simulink model "eovsa_corr_300mhz"  (R2012b)
settings: Solver=VariableStepDiscrete  SolverMode=SingleTasking  StartTime=0.0  StopTime=5000  RelTol=1e-3
undefined symbols (not defined in the file or in its folder): A, B, gcbh, PCIN, sfp, xlBlockLoadCallback, xlipgetpartsetting
libraries: xbsIndex_r4 x5996, casper_library_misc x52, simulink x33, dspsigops x24, xps_library x15, casper_library_delays x2
(part 6 of 65)

== system eovsa_corr_300mhz/packet_buffer0 ==
  note: TODO: Clean up some no longer used logic.
  din : Inport
  dvalid : Inport  Port=2
  eof : Inport  Port=3
  hdr : Inport  Port=4
  hdr_valid : Inport  Port=5
  rd_addr_in : Inport  Port=6
  rd_valid_in : Inport  Port=7
  Convert3 : xbsIndex_r4/Convert  gui_display_data_type=Fixed-point  arith_type=Unsigned  n_bits=n_boards  bin_pt=0  float_type=Single  exp_bits=8  fraction_bits=24  quantization=Truncate  overflow=Wrap  en=off  latency=0  dbl_ovrd=off  pipeline=off  block_type=convert
      settings: block_version=11.4
  Delay{1,3,5,7..10,15..17,19..20,22..25} (16 alike) : xbsIndex_r4/Delay  rst=off  infoeditControl=Selection of Reset will increase slice count due to use of real FFs and instead of SRLs  en=off  latency=1  dbl_ovrd=off  reg_retiming=on  block_type=delay
      settings: block_version=11.4
  Delay4 : xbsIndex_r4/Delay  rst=off  infoeditControl=Selection of Reset will increase slice count due to use of real FFs and instead of SRLs  en=on  latency=1  dbl_ovrd=off  reg_retiming=on  block_type=delay
      settings: block_version=11.4
  Logical : xbsIndex_r4/Logical  logical_function=AND  inputs=2  en=off  latency=0  precision=Full  arith_type=Unsigned  n_bits=16  bin_pt=0  align_bp=on  dbl_ovrd=off  block_type=logical
  Slice1 : xbsIndex_r4/Slice  nbits=16  boolean_output=off  mode=Lower Bit Location + Width  bit1=0  base1=MSB of Input  bit0=0  base0=LSB of Input  dbl_ovrd=off  block_type=slice
  Slice3 : xbsIndex_r4/Slice  nbits=48  boolean_output=off  mode=Upper Bit Location + Width  bit1=0  base1=MSB of Input  bit0=0  base0=LSB of Input  dbl_ovrd=off  block_type=slice
  Slice5 : xbsIndex_r4/Slice  nbits=freq_chan - (n_boards + n_x)  boolean_output=off  mode=Lower Bit Location + Width  bit1=0  base1=MSB of Input  bit0=16  base0=LSB of Input  dbl_ovrd=off  block_type=slice
  buffer0 : Subsystem
  word_counter : xbsIndex_r4/Counter  cnt_type=Free Running  cnt_to=Inf  operation=Up  start_count=0  cnt_by_val=1  arith_type=Unsigned  n_bits=pkt_len  bin_pt=0  load_pin=off  rst=on  en=on  explicit_period=off  period=1  dbl_ovrd=off  use_behavioral_HDL=off  implementation=Fabric  block_type=counter
      settings: block_version=11.4
  sync : Outport
  d0 : Outport  Port=2
  dv0 : Outport  Port=3
  mcnt_out0 : Outport  Port=4
  rd_addr_out : Outport  Port=5
  rd_valid_out0 : Outport  Port=6
  rd_valid_out1 : Outport  Port=7
  wires:
  Delay15/1 -> [din]
  Delay9/1 -> [word]
  Delay8/1 -> [ant]
  Delay5/1 -> [freq]
  Delay3/1 -> [we]
  Delay1/1 -> [mcnt]
  Convert3/1 -> Delay22/1
  Delay23/1 -> Delay1/1
  Slice5/1 -> Delay16/1
  Delay22/1 -> Delay8/1
  Delay17/1 -> Delay9/1
  Delay16/1 -> Delay5/1
  Delay10/1 -> Delay15/1
  din/1 -> Delay10/1
  Delay7/1 -> Delay3/1
  hdr_valid/1 -> Delay4/2
  Delay4/1 -> Slice5/1, Slice3/1, Slice1/1
  hdr/1 -> Delay4/1
  dvalid/1 -> Logical/1, word_counter/2, Delay7/1
  buffer0/4(mcnt) -> mcnt_out0/1
  buffer0/3(dout_valid) -> dv0/1
  buffer0/2(dout) -> d0/1
  buffer0/1(sync) -> sync/1
  word_counter/1 -> Delay17/1
  Slice3/1 -> Delay23/1
  Slice1/1 -> Convert3/1
  [din] -> buffer0/1(data)
  [freq] -> buffer0/2(freq)
  [we] -> buffer0/3(dvalid)
  [ant] -> buffer0/4(ant)
  [word] -> buffer0/5(word)
  [mcnt] -> buffer0/6(mcnt_in)
  buffer0/6(rd_valid_out0) -> rd_valid_out0/1
  buffer0/5(rd_addr_out) -> rd_addr_out/1
  Delay20/1 -> [rd_addr_in]
  Delay19/1 -> Delay20/1
  Delay25/1 -> [rd_valid_in]
  Delay24/1 -> Delay25/1
  rd_addr_in/1 -> Delay19/1
  rd_valid_in/1 -> Delay24/1
  [rd_addr_in] -> buffer0/7(rd_addr_in)
  [rd_valid_in] -> buffer0/8(rd_valid_in)
  Logical/1 -> word_counter/1
  eof/1 -> Logical/2
  buffer0/7(rd_valid_out1) -> rd_valid_out1/1

== system eovsa_corr_300mhz/packet_buffer1 ==
  note: TODO: Clean up some no longer used logic.
  din : Inport
  dvalid : Inport  Port=2
  eof : Inport  Port=3
  hdr : Inport  Port=4
  hdr_valid : Inport  Port=5
  rd_addr_in : Inport  Port=6
  rd_valid_in : Inport  Port=7
  Convert3 : xbsIndex_r4/Convert  gui_display_data_type=Fixed-point  arith_type=Unsigned  n_bits=n_boards  bin_pt=0  float_type=Single  exp_bits=8  fraction_bits=24  quantization=Truncate  overflow=Wrap  en=off  latency=0  dbl_ovrd=off  pipeline=off  block_type=convert
      settings: block_version=11.4
  Delay{1,3,5,7..10,15..17,19..20,22..25} (16 alike) : xbsIndex_r4/Delay  rst=off  infoeditControl=Selection of Reset will increase slice count due to use of real FFs and instead of SRLs  en=off  latency=1  dbl_ovrd=off  reg_retiming=on  block_type=delay
      settings: block_version=11.4
  Delay4 : xbsIndex_r4/Delay  rst=off  infoeditControl=Selection of Reset will increase slice count due to use of real FFs and instead of SRLs  en=on  latency=1  dbl_ovrd=off  reg_retiming=on  block_type=delay
      settings: block_version=11.4
  Logical : xbsIndex_r4/Logical  logical_function=AND  inputs=2  en=off  latency=0  precision=Full  arith_type=Unsigned  n_bits=16  bin_pt=0  align_bp=on  dbl_ovrd=off  block_type=logical
  Slice1 : xbsIndex_r4/Slice  nbits=16  boolean_output=off  mode=Lower Bit Location + Width  bit1=0  base1=MSB of Input  bit0=0  base0=LSB of Input  dbl_ovrd=off  block_type=slice
  Slice3 : xbsIndex_r4/Slice  nbits=48  boolean_output=off  mode=Upper Bit Location + Width  bit1=0  base1=MSB of Input  bit0=0  base0=LSB of Input  dbl_ovrd=off  block_type=slice
  Slice5 : xbsIndex_r4/Slice  nbits=freq_chan - (n_boards + n_x)  boolean_output=off  mode=Lower Bit Location + Width  bit1=0  base1=MSB of Input  bit0=16  base0=LSB of Input  dbl_ovrd=off  block_type=slice
  buffer0 : Subsystem
  word_counter : xbsIndex_r4/Counter  cnt_type=Free Running  cnt_to=Inf  operation=Up  start_count=0  cnt_by_val=1  arith_type=Unsigned  n_bits=pkt_len  bin_pt=0  load_pin=off  rst=on  en=on  explicit_period=off  period=1  dbl_ovrd=off  use_behavioral_HDL=off  implementation=Fabric  block_type=counter
      settings: block_version=11.4
  sync : Outport
  d0 : Outport  Port=2
  dv0 : Outport  Port=3
  mcnt_out0 : Outport  Port=4
  rd_addr_out : Outport  Port=5
  rd_valid_out0 : Outport  Port=6
  rd_valid_out1 : Outport  Port=7
  wires:
  buffer0/7(rd_valid_out1) -> rd_valid_out1/1
  eof/1 -> Logical/2
  Logical/1 -> word_counter/1
  [rd_valid_in] -> buffer0/8(rd_valid_in)
  [rd_addr_in] -> buffer0/7(rd_addr_in)
  rd_valid_in/1 -> Delay24/1
  rd_addr_in/1 -> Delay19/1
  Delay24/1 -> Delay25/1
  Delay25/1 -> [rd_valid_in]
  Delay19/1 -> Delay20/1
  Delay20/1 -> [rd_addr_in]
  buffer0/5(rd_addr_out) -> rd_addr_out/1
  buffer0/6(rd_valid_out0) -> rd_valid_out0/1
  [mcnt] -> buffer0/6(mcnt_in)
  [word] -> buffer0/5(word)
  [ant] -> buffer0/4(ant)
  [we] -> buffer0/3(dvalid)
  [freq] -> buffer0/2(freq)
  [din] -> buffer0/1(data)
  Slice1/1 -> Convert3/1
  Slice3/1 -> Delay23/1
  word_counter/1 -> Delay17/1
  buffer0/1(sync) -> sync/1
  buffer0/2(dout) -> d0/1
  buffer0/3(dout_valid) -> dv0/1
  buffer0/4(mcnt) -> mcnt_out0/1
  dvalid/1 -> Delay7/1, word_counter/2, Logical/1
  hdr/1 -> Delay4/1
  Delay4/1 -> Slice1/1, Slice3/1, Slice5/1
  hdr_valid/1 -> Delay4/2
  Delay7/1 -> Delay3/1
  din/1 -> Delay10/1
  Delay10/1 -> Delay15/1
  Delay16/1 -> Delay5/1
  Delay17/1 -> Delay9/1
  Delay22/1 -> Delay8/1
  Slice5/1 -> Delay16/1
  Delay23/1 -> Delay1/1
  Convert3/1 -> Delay22/1
  Delay1/1 -> [mcnt]
  Delay3/1 -> [we]
  Delay5/1 -> [freq]
  Delay8/1 -> [ant]
  Delay9/1 -> [word]
  Delay15/1 -> [din]

== system eovsa_corr_300mhz/packet_count_p ==
  out_reg : Inport
  assert_reg : xbsIndex_r4/Assert  assert_type=on  type_source=Explicitly  gui_display_data_type=Fixed-point  arith_type=Unsigned  n_bits=32  bin_pt=0  preci_type=Single  exp_width=8  frac_width=24  assert_rate=off  rate_source=Explicitly  period=1  output_port=on  block_type=assert
  cast_gw : xbsIndex_r4/Convert  gui_display_data_type=Fixed-point  arith_type=Unsigned  n_bits=32  bin_pt=0  float_type=Single  exp_bits=8  fraction_bits=24  quantization=Truncate  overflow=Wrap  en=off  latency=0  dbl_ovrd=off  pipeline=off  block_type=convert
  eovsa_corr_300mhz_packet_count_p_user_data_in : xbsIndex_r4/Gateway Out  inherit_from_input=off  hdl_port=on  timing_constraint=None  locs_specified=off  LOCs={}  UseAsDAC=off  DACChannel='1'  block_type=gatewayout
  io_delay : xbsIndex_r4/Delay  rst=off  infoeditControl=Selection of Reset will increase slice count due to use of real FFs and instead of SRLs  en=off  latency=0  dbl_ovrd=off  reg_retiming=on  block_type=delay
  reint1 : xbsIndex_r4/Reinterpret  force_arith_type=on  arith_type=Unsigned  force_bin_pt=on  bin_pt=0  block_type=reinterpret
  sim_out : Outport
  wires:
  io_delay/1 -> cast_gw/1
  cast_gw/1 -> eovsa_corr_300mhz_packet_count_p_user_data_in/1
  eovsa_corr_300mhz_packet_count_p_user_data_in/1 -> sim_out/1
  out_reg/1 -> assert_reg/1
  assert_reg/1 -> reint1/1
  reint1/1 -> io_delay/1

== system eovsa_corr_300mhz/packet_count_x ==
  out_reg : Inport
  assert_reg : xbsIndex_r4/Assert  assert_type=on  type_source=Explicitly  gui_display_data_type=Fixed-point  arith_type=Unsigned  n_bits=32  bin_pt=0  preci_type=Single  exp_width=8  frac_width=24  assert_rate=off  rate_source=Explicitly  period=1  output_port=on  block_type=assert
  cast_gw : xbsIndex_r4/Convert  gui_display_data_type=Fixed-point  arith_type=Unsigned  n_bits=32  bin_pt=0  float_type=Single  exp_bits=8  fraction_bits=24  quantization=Truncate  overflow=Wrap  en=off  latency=0  dbl_ovrd=off  pipeline=off  block_type=convert
  eovsa_corr_300mhz_packet_count_x_user_data_in : xbsIndex_r4/Gateway Out  inherit_from_input=off  hdl_port=on  timing_constraint=None  locs_specified=off  LOCs={}  UseAsDAC=off  DACChannel='1'  block_type=gatewayout
  io_delay : xbsIndex_r4/Delay  rst=off  infoeditControl=Selection of Reset will increase slice count due to use of real FFs and instead of SRLs  en=off  latency=0  dbl_ovrd=off  reg_retiming=on  block_type=delay
  reint1 : xbsIndex_r4/Reinterpret  force_arith_type=on  arith_type=Unsigned  force_bin_pt=on  bin_pt=0  block_type=reinterpret
  sim_out : Outport
  wires:
  io_delay/1 -> cast_gw/1
  cast_gw/1 -> eovsa_corr_300mhz_packet_count_x_user_data_in/1
  eovsa_corr_300mhz_packet_count_x_user_data_in/1 -> sim_out/1
  out_reg/1 -> assert_reg/1
  assert_reg/1 -> reint1/1
  reint1/1 -> io_delay/1

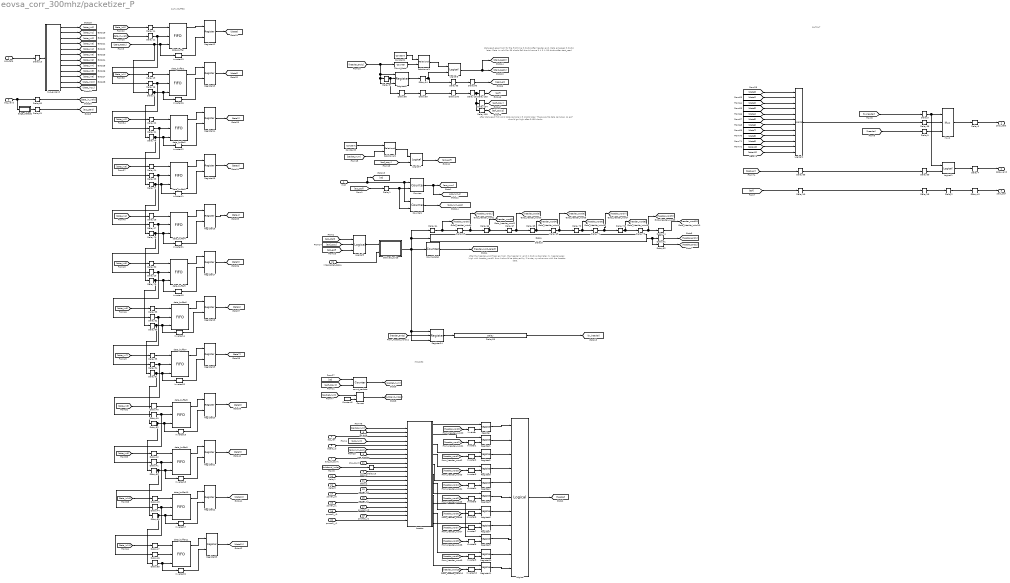
== system eovsa_corr_300mhz/packetizer_P ==
  note: After the header_word flags go high, the header is valid 2 clock cycles later.
      | tx_header goes high with header_word0, thus it should be delayed by 2 to stay synchronous with the header data.
  note: after start_read first valid data sample is 3 clocks later.
      | There are 96 data samples, so eof should go high after 3+95 clocks
  note: start_read goes high for the first time 3 clocks after header_end.
      | Data emerges 3 clocks later.
      | Data is valid for 96 clocks
      | Eof should come 3 + 3 + 95 clocks after start_read
  note: OUTPUT
  note: HEADER
  note: DATA BUFFER
  mrst : Inport
  acc_data : Inport  Port=2
  acc_valid : Inport  Port=3
  acc_len : Inport  Port=4
  use_circular : Inport  Port=5
  board_id : Inport  Port=6
  adc_of_count : Inport  Port=7
  fft_shift : Inport  Port=8
  delay0 : Inport  Port=9
  delay1 : Inport  Port=10
  delay2 : Inport  Port=11
  delay3 : Inport  Port=12
  power_x0 : Inport  Port=13
  power_y0 : Inport  Port=14
  power_x1 : Inport  Port=15
  power_y1 : Inport  Port=16
  power2_x0 : Inport  Port=17
  power2_y0 : Inport  Port=18
  power2_x1 : Inport  Port=19
  power2_y1 : Inport  Port=20
  clip_count : Inport  Port=21
  interpacket_delay : Inport  Port=22
  Concat : xbsIndex_r4/Concat  num_inputs=2  dbl_ovrd=off  block_type=concat
  Constant1 : xbsIndex_r4/Constant  const=0  gui_display_data_type=Fixed-point  arith_type=Unsigned  n_bits=4  bin_pt=0  preci_type=Single  exp_width=8  frac_width=24  explicit_period=on  period=1  equ=P=C  opselect=C  inp2=PCIN>>17  opr=+  inp1=P  carry=CIN  dbl_ovrd=off  block_type=constant
      settings: block_version=11.4
  Constant2 : xbsIndex_r4/Constant  const=0  gui_display_data_type=Fixed-point  arith_type=Unsigned  n_bits=log2( (2 ^ freq_chan) / n_packets )  bin_pt=0  preci_type=Single  exp_width=8  frac_width=24  explicit_period=on  period=1  equ=P=C  opselect=C  inp2=PCIN>>17  opr=+  inp1=P  carry=CIN  dbl_ovrd=off  block_type=constant
      settings: block_version=11.4
  Constant3 : xbsIndex_r4/Constant  const=n_packets - 1  gui_display_data_type=Fixed-point  arith_type=Unsigned  n_bits=ceil( log2( n_packets - 1 ) )  bin_pt=0  preci_type=Single  exp_width=8  frac_width=24  explicit_period=on  period=1  equ=P=C  opselect=C  inp2=PCIN>>17  opr=+  inp1=P  carry=CIN  dbl_ovrd=off  block_type=constant
      settings: block_version=11.4
  Count_data1 : xbsIndex_r4/Counter  cnt_type=Count Limited  cnt_to=header_len / 8 - 1  operation=Up  start_count=0  cnt_by_val=1  arith_type=Unsigned  n_bits=ceil( log2( header_len / 8 - 1 ) )  bin_pt=0  load_pin=off  rst=on  en=off  explicit_period=on  period=1  dbl_ovrd=off  use_behavioral_HDL=on  implementation=Fabric  use_rpm=off  block_type=counter
  Count_data7 : xbsIndex_r4/Counter  cnt_type=Count Limited  cnt_to=11  operation=Up  start_count=0  cnt_by_val=1  arith_type=Unsigned  n_bits=4  bin_pt=0  load_pin=off  rst=on  en=off  explicit_period=on  period=1  dbl_ovrd=off  use_behavioral_HDL=on  implementation=Fabric  use_rpm=off  block_type=counter
  Counter : xbsIndex_r4/Counter  cnt_type=Free Running  cnt_to=Inf  operation=Up  start_count=0  cnt_by_val=1  arith_type=Unsigned  n_bits=32  bin_pt=0  load_pin=off  rst=on  en=on  explicit_period=off  period=1  dbl_ovrd=off  use_behavioral_HDL=off  implementation=DSP48  block_type=counter
      settings: block_version=11.4
  Counter1 : xbsIndex_r4/Counter  cnt_type=Count Limited  cnt_to=49  operation=Up  start_count=0  cnt_by_val=1  arith_type=Unsigned  n_bits=8  bin_pt=0  load_pin=off  rst=on  en=on  explicit_period=off  period=1  dbl_ovrd=off  use_behavioral_HDL=off  implementation=Fabric  block_type=counter
      settings: block_version=11.4
  Delay{1..4,6,9,13..14,32,34,41,43..44,48..49,56,58..59,64..74,95,98..100} (33 alike) : xbsIndex_r4/Delay  rst=off  infoeditControl=Selection of Reset will increase slice count due to use of real FFs and instead of SRLs  en=off  latency=1  dbl_ovrd=off  reg_retiming=on  block_type=delay
      settings: block_version=11.4
  Delay{7,11,15..16,21,23,27,29,39,46,60..61,76..85,91..92,94,102..105} (29 alike) : xbsIndex_r4/Delay  rst=off  infoeditControl=Selection of Reset will increase slice count due to use of real FFs and instead of SRLs  en=off  latency=1  dbl_ovrd=off  reg_retiming=off  block_type=delay
      settings: block_version=11.4
  Delay19 : xbsIndex_r4/Delay  rst=off  infoeditControl=Selection of Reset will increase slice count due to use of real FFs and instead of SRLs  en=off  latency=2  dbl_ovrd=off  reg_retiming=on  block_type=delay
      settings: block_version=11.4
  Delay22 : xbsIndex_r4/Delay  rst=off  infoeditControl=Selection of Reset will increase slice count due to use of real FFs and instead of SRLs  en=off  latency=3  dbl_ovrd=off  reg_retiming=on  block_type=delay
      settings: block_version=11.4
  Delay24 : xbsIndex_r4/Delay  rst=off  infoeditControl=Selection of Reset will increase slice count due to use of real FFs and instead of SRLs  en=off  latency=4  dbl_ovrd=off  reg_retiming=on  block_type=delay
      settings: block_version=11.4
  Delay28 : xbsIndex_r4/Delay  rst=off  infoeditControl=Selection of Reset will increase slice count due to use of real FFs and instead of SRLs  en=off  latency=5  dbl_ovrd=off  reg_retiming=on  block_type=delay
      settings: block_version=11.4
  Delay30 : xbsIndex_r4/Delay  rst=off  infoeditControl=Selection of Reset will increase slice count due to use of real FFs and instead of SRLs  en=off  latency=6  dbl_ovrd=off  reg_retiming=on  block_type=delay
      settings: block_version=11.4
  Delay33 : xbsIndex_r4/Delay  rst=off  infoeditControl=Selection of Reset will increase slice count due to use of real FFs and instead of SRLs  en=off  latency=7  dbl_ovrd=off  reg_retiming=on  block_type=delay
      settings: block_version=11.4
  Delay35 : xbsIndex_r4/Delay  rst=off  infoeditControl=Selection of Reset will increase slice count due to use of real FFs and instead of SRLs  en=off  latency=8  dbl_ovrd=off  reg_retiming=on  block_type=delay
      settings: block_version=11.4
  Delay40 : xbsIndex_r4/Delay  rst=off  infoeditControl=Selection of Reset will increase slice count due to use of real FFs and instead of SRLs  en=off  latency=9  dbl_ovrd=off  reg_retiming=on  block_type=delay
      settings: block_version=11.4
  Delay42 : xbsIndex_r4/Delay  rst=off  infoeditControl=Selection of Reset will increase slice count due to use of real FFs and instead of SRLs  en=off  latency=10  dbl_ovrd=off  reg_retiming=on  block_type=delay
      settings: block_version=11.4
  Delay45 : xbsIndex_r4/Delay  rst=off  infoeditControl=Selection of Reset will increase slice count due to use of real FFs and instead of SRLs  en=off  latency=11  dbl_ovrd=off  reg_retiming=on  block_type=delay
      settings: block_version=11.4
  Delay47 : xbsIndex_r4/Delay  rst=off  infoeditControl=Selection of Reset will increase slice count due to use of real FFs and instead of SRLs  en=off  latency=12  dbl_ovrd=off  reg_retiming=on  block_type=delay
      settings: block_version=11.4
  Delay5 : xbsIndex_r4/Delay  rst=off  infoeditControl=Selection of Reset will increase slice count due to use of real FFs and instead of SRLs  en=off  latency=10  dbl_ovrd=off  reg_retiming=on  block_type=delay
      settings: block_version=11.4
  Delay53 : xbsIndex_r4/Delay  rst=off  infoeditControl=Selection of Reset will increase slice count due to use of real FFs and instead of SRLs  en=off  latency=2  dbl_ovrd=off  reg_retiming=on  block_type=delay
      settings: block_version=11.4
  Delay96 : xbsIndex_r4/Delay  rst=off  infoeditControl=Selection of Reset will increase slice count due to use of real FFs and instead of SRLs  en=off  latency=3  dbl_ovrd=off  reg_retiming=on  block_type=delay
      settings: block_version=11.4
  Delay97 : xbsIndex_r4/Delay  rst=off  infoeditControl=Selection of Reset will increase slice count due to use of real FFs and instead of SRLs  en=off  latency=data_len / 8  dbl_ovrd=off  reg_retiming=off  block_type=delay
      settings: block_version=11.4
  Inverter{,1..10} (11 alike) : xbsIndex_r4/Inverter  en=off  latency=0  dbl_ovrd=off  block_type=inv
  Inverter{11..22} (12 alike) : xbsIndex_r4/Inverter  en=off  latency=2  dbl_ovrd=off  block_type=inv
  Logical : xbsIndex_r4/Logical  logical_function=OR  inputs=11  en=off  latency=1  precision=Full  arith_type=Unsigned  n_bits=16  bin_pt=0  align_bp=on  dbl_ovrd=off  block_type=logical
  Logical1 : xbsIndex_r4/Logical  logical_function=OR  inputs=2  en=off  latency=1  precision=Full  arith_type=Unsigned  n_bits=16  bin_pt=0  align_bp=on  dbl_ovrd=off  block_type=logical
      settings: block_version=11.4
  Logical2 : xbsIndex_r4/Logical  logical_function=OR  inputs=12  en=off  latency=1  precision=Full  arith_type=Unsigned  n_bits=16  bin_pt=0  align_bp=on  dbl_ovrd=off  block_type=logical
  Logical4 : xbsIndex_r4/Logical  logical_function=AND  inputs=2  en=off  latency=0  precision=Full  arith_type=Unsigned  n_bits=16  bin_pt=0  align_bp=on  dbl_ovrd=off  block_type=logical
      settings: block_version=11.4
  Logical5 : xbsIndex_r4/Logical  logical_function=AND  inputs=2  en=off  latency=1  precision=Full  arith_type=Unsigned  n_bits=16  bin_pt=0  align_bp=on  dbl_ovrd=off  block_type=logical
      settings: block_version=11.4
  Logical9 : xbsIndex_r4/Logical  logical_function=XOR  inputs=3  en=off  latency=0  precision=Full  arith_type=Unsigned  n_bits=16  bin_pt=0  align_bp=on  dbl_ovrd=off  block_type=logical
      settings: block_version=11.4
  Mux2 : xbsIndex_r4/Mux  inputs=2  en=off  latency=1  precision=Full  arith_type=Unsigned  n_bits=16  bin_pt=14  quantization=Truncate  overflow=Wrap  dbl_ovrd=off  block_type=mux
      settings: block_version=11.4
  Register{,1..7,9..23} (23 alike) : xbsIndex_r4/Register  init=0  rst=on  en=off  dbl_ovrd=off  block_type=register
  Register24 : xbsIndex_r4/Register  init=0  rst=on  en=on  dbl_ovrd=off  block_type=register
  Register8 : xbsIndex_r4/Register  init=0  rst=on  en=on  dbl_ovrd=off  block_type=register
  Relational1 : xbsIndex_r4/Relational  mode=a=b  en=off  latency=1  dbl_ovrd=off  block_type=relational
  Relational2 : xbsIndex_r4/Relational  mode=a=b  en=off  latency=1  dbl_ovrd=off  block_type=relational
  bus_expand : Subsystem  AncestorBlock=casper_library_flow_control/bus_expand  mask(bus_expand){mode=divisions of equal size, outputNum=12, outputWidth=64, outputBinaryPt=0, outputArithmeticType=0, show_format=off, outputToWorkspace=off, variablePrefix=out, outputToModelAsWell=on}
      mask prompts: outputNum "Number of outputs:"; outputWidth "Output width:"; outputBinaryPt "Output binary point position:"; outputArithmeticType "Output arithmetic type (ufix=0, fix=1, bool=2):"; show_format "Print format string?"; outputToWorkspace "Output to workspace?"; variablePrefix "Variable name prefix:"; outputToModelAsWell "Output to model as well?"
      mask help:
      | Expands a 'bus' made using a bus_create or Xilinx
      | concat block.
      | The input will be divided into the specified number
      | of outputs with the specified arithmetic types.
      | Divisions are made from most significant bit.
      mask init: same as eovsa_corr_300mhz/bus_expand7
      settings: AttributesFormatString=12 outputs
      mask TypeOptions mode: divisions of equal size | divisions of arbitrary size
      mask Callback mode: bus_expand_callback();
      mask Callback outputWidth: bus_expand_callback();
      mask Callback outputToWorkspace: bus_expand_callback();
  count_packets : xbsIndex_r4/Counter  cnt_type=Count Limited  cnt_to=n_packets - 1  operation=Up  start_count=0  cnt_by_val=1  arith_type=Unsigned  n_bits=ceil( log2( n_packets ) )  bin_pt=0  load_pin=off  rst=on  en=on  explicit_period=off  period=1  dbl_ovrd=off  use_behavioral_HDL=off  implementation=DSP48  use_rpm=off  block_type=counter
  data_buffer{,1..11} (12 alike) : xbsIndex_r4/FIFO  mem_type=Block RAM  performance_options=Standard_FIFO  infoedit1=Available only for V4, V5, V6, V7, K7, A7 and Zynq devices.  embedded_registers=on  depth=2K  percent_nbits=1  rst=off  en=off  use_dcount=off  use_percent_full_port=off  use_almost_empty=off  almost_empty_thresh=2  use_almost_full=off  almost_full_thresh=14  dbl_ovrd=off  explicit_period=off  block_type=fifo
      settings: block_version=10.1.3
  delayed_pulse : Subsystem
  edge_detect2 : Subsystem  AncestorBlock=casper_library_misc/edge_detect  mask(edge_detect){edge=Rising, polarity=Active High, x_in=[0 0.08 0.08 0.16 0.16 0.24 0.24 0.32 0.32 0.4], y_in=[-1 -1  1  1  1  1  1  1  1  1], x_out=[0.6 0.68 0.68 0.76 0.76 0.84 0.84 0.92 0.92 1], y_out=[-1 -1  1  1 -1 -1 -1 -1 -1 -1]}
      mask prompts: edge "Edge Type"; polarity "Output Polarity"; x_in "Input X Positions"; y_in "Input Y Positions"; x_out "Output X Positions"; y_out "Output Y Positions"
      mask help: Output is active for one-cycle after each edge of the specified type (i.e. rising, falling or both).
      mask init: same as eovsa_corr_300mhz/edge_detect1
      settings: AttributesFormatString=|
      | rising edges
      | active high
      mask Help: Output is active for one-cycle after each edge of the specified type (i.e. rising, falling, or both).  Latency is zero.
      mask TypeOptions edge: Rising | Falling | Both
      mask TypeOptions polarity: Active High | Active Low
      mask Display:
      | plot(x_in_num,0.5+y_in_num*0.2);
      | plot(x_out_num,0.5+y_out_num*0.2);
  header : Subsystem
  pack_data : Outport
  data_valid : Outport  Port=2
  pack_eof : Outport  Port=3
  tag scope: acc_num_P=global
  wires:
  Delay14/1 -> data_buffer/1
  Delay11/1 -> Delay16/1, data_buffer/2
  acc_data/1 -> Delay13/1
  Mux2/1 -> Delay6/1
  [eof_copy] -> Logical9/2
  [acc_start] -> Logical9/1
  Count_data1/1 -> [header_word_select]
  Logical1/1 -> Delay4/1
  edge_detect2/1(out) -> Delay61/1
  acc_len/1 -> header/3(acc_len)
  [acc_num] -> header/4(acc_num)
  [acc_num_pps] -> header/6(acc_num_pps)
  use_circular/1 -> header/7(circular)
  Constant3/1 -> Relational2/1
  [packet_num] -> Relational2/2
  Relational2/1 -> Logical4/1
  Logical4/1 -> [acc_eof]
  [acc_eof] -> Logical9/3
  adc_of_count/1 -> header/8(adc_of_count)
  Constant2/1 -> Concat/2
  Concat/1 -> [subband_index]
  [subband_index] -> Delay15/1
  fft_shift/1 -> header/2(fft_shift)
  delay0/1 -> header/11(delay0)
  delay1/1 -> header/12(delay1)
  delay2/1 -> header/13(delay2)
  delay3/1 -> header/14(delay3)
  power_x0/1 -> header/15(power_x0)
  power_y0/1 -> header/16(power_y0)
  power_y1/1 -> header/18(power_y1)
  power_x1/1 -> header/17(power_x1)
  power2_x0/1 -> header/19(power2_x0)
  power2_y0/1 -> header/20(power2_y0)
  power2_x1/1 -> header/21(power2_x1)
  power2_y1/1 -> header/22(power2_y1)
  [data0] -> Logical2/1
  Delay56/1 -> Delay59/1
  [eof_copy] -> Logical4/2
  clip_count/1 -> header/9(clip_count)
  Delay3/1 -> Logical1/1, Mux2/1
  Logical/1 -> [header]
  Delay4/1 -> data_valid/1
  Delay6/1 -> pack_data/1
  interpacket_delay/1 -> delayed_pulse/2(In2)
  delayed_pulse/1(delayed_eof) -> Register24/1, Register24/3, Delay5/1, Delay64/1, Count_data1/1
  Logical9/1 -> delayed_pulse/1(pack_eof)
  mrst/1 -> Counter/1, Counter1/1, [rst]
  Delay1/1 -> Counter/2, Counter1/2
  Counter1/1 -> [acc_num_pps]
  [acc_eof] -> Delay1/1
  [eof_copy2] -> count_packets/2
  [rst] -> count_packets/1
  [tx_header] -> Delay3/1
  Delay9/1 -> Mux2/3
  bus_expand/1(msb_out12) -> [data_in0]
  bus_expand/2(out11) -> [data_in1]
  bus_expand/3(out10) -> [data_in2]
  bus_expand/4(out9) -> [data_in3]
  bus_expand/5(out8) -> [data_in4]
  bus_expand/6(out7) -> [data_in5]
  bus_expand/7(out6) -> [data_in6]
  bus_expand/8(out5) -> [data_in7]
  bus_expand/9(out4) -> [data_in8]
  bus_expand/10(out3) -> [data_in9]
  bus_expand/11(out2) -> [data_in10]
  bus_expand/12(lsb_out1) -> [data_in11]
  Delay13/1 -> bus_expand/1(bus_in)
  acc_valid/1 -> Delay60/1, edge_detect2/1(in)
  [data_in0] -> Delay14/1
  [data_in_valid] -> Delay11/1
  Delay19/1 -> data_buffer1/1
  Delay16/1 -> Delay21/1, data_buffer1/2
  [data_in1] -> Delay19/1
  Delay22/1 -> data_buffer2/1
  Delay21/1 -> Delay23/1, data_buffer2/2
  [data_in2] -> Delay22/1
  Delay24/1 -> data_buffer3/1
  Delay23/1 -> Delay27/1, data_buffer3/2
  [data_in3] -> Delay24/1
  Delay28/1 -> data_buffer4/1
  Delay27/1 -> Delay29/1, data_buffer4/2
  [data_in4] -> Delay28/1
  Delay30/1 -> data_buffer5/1
  Delay29/1 -> Delay32/1, data_buffer5/2
  [data_in5] -> Delay30/1
  Delay33/1 -> data_buffer6/1
  Delay32/1 -> Delay34/1, data_buffer6/2
  [data_in6] -> Delay33/1
  Delay35/1 -> data_buffer7/1
  Delay34/1 -> Delay39/1, data_buffer7/2
  [data_in7] -> Delay35/1
  Delay40/1 -> data_buffer8/1
  Delay39/1 -> data_buffer8/2, Delay41/1
  [data_in8] -> Delay40/1
  Delay42/1 -> data_buffer9/1
  Delay41/1 -> data_buffer9/2, Delay44/1
  [data_in9] -> Delay42/1
  Delay45/1 -> data_buffer10/1
  Delay44/1 -> data_buffer10/2, Delay46/1
  Delay84/1 -> Delay85/1, Inverter17/1, data_buffer10/3
  [data_in10] -> Delay45/1
  Delay47/1 -> data_buffer11/1
  Delay46/1 -> data_buffer11/2
  [data_in11] -> Delay47/1
  [data1] -> Logical2/2
  [data2] -> Logical2/3
  [data3] -> Logical2/4
  [data4] -> Logical2/5
  [data5] -> Logical2/6
  [data6] -> Logical2/7
  [data7] -> Logical2/8
  [data8] -> Logical2/9
  [data9] -> Logical2/10
  [data10] -> Logical2/11
  [data11] -> Logical2/12
  count_packets/1 -> [packet_num]
  [packet_num] -> header/1(packet_num)
  [packet_num] -> Concat/1
  Delay2/1 -> Delay43/1
  Logical2/1 -> Delay58/1
  [read_en] -> Delay56/1
  [header] -> Delay9/1
  Delay58/1 -> Mux2/2
  Delay59/1 -> Logical1/2
  board_id/1 -> header/5(board_id)
  Counter/1 -> [acc_num_P], [acc_num]
  Delay60/1 -> [data_in_valid]
  Delay61/1 -> [acc_start]
  Delay15/1 -> header/10(subband_index)
  Delay64/1 -> Delay65/1, [header_word0]
  Delay65/1 -> Delay66/1, [header_word1]
  Delay66/1 -> [header_word2], Delay67/1
  Delay67/1 -> [header_word3], Delay68/1
  Delay68/1 -> [header_word4], Delay69/1
  Delay69/1 -> [header_word5], Delay70/1
  Delay70/1 -> [header_word6], Delay71/1
  Delay71/1 -> [header_word7], Delay72/1
  [header_word0] -> Inverter/1
  [header_word1] -> Inverter1/1
  [header_word2] -> Inverter2/1
  [header_word3] -> Inverter3/1
  [header_word4] -> Inverter4/1
  [header_word5] -> Inverter5/1
  [header_word6] -> Inverter6/1
  [header_word7] -> Inverter7/1
  Inverter/1 -> Register/2
  Inverter1/1 -> Register1/2
  Inverter2/1 -> Register2/2
  Inverter3/1 -> Register3/2
  Inverter4/1 -> Register4/2
  Inverter5/1 -> Register5/2
  Inverter6/1 -> Register6/2
  Inverter7/1 -> Register7/2
  header/1(header0) -> Register/1
  header/2(header1) -> Register1/1
  header/3(header2) -> Register2/1
  header/4(header3) -> Register3/1
  header/5(header4) -> Register4/1
  header/6(header5) -> Register5/1
  header/7(header6) -> Register6/1
  header/8(header7) -> Register7/1
  Delay72/1 -> [header_word8], Delay73/1
  Delay73/1 -> [header_word9], Delay74/1
  Register24/1 -> Delay53/1
  Delay74/1 -> [header_word10]
  [header_word8] -> Inverter8/1
  Inverter8/1 -> Register9/2
  [header_word9] -> Inverter9/1
  Inverter9/1 -> Register10/2
  [header_word10] -> Inverter10/1
  Inverter10/1 -> Register11/2
  header/9(header8) -> Register9/1
  header/10(header9) -> Register10/1
  header/11(header10) -> Register11/1
  Register9/1 -> Logical/9
  Register11/1 -> Logical/11
  Register5/1 -> Logical/6
  Register4/1 -> Logical/5
  Register2/1 -> Logical/3
  Register3/1 -> Logical/4
  Register6/1 -> Logical/7
  Register10/1 -> Logical/10
  Register7/1 -> Logical/8
  Register1/1 -> Logical/2
  Register/1 -> Logical/1
  Delay5/1 -> Delay92/1, Delay91/1
  [start_read1] -> Delay7/1, Inverter13/1, data_buffer/3
  Register12/1 -> [data0]
  Inverter13/1 -> Register12/2
  Delay7/1 -> Delay76/1, Inverter16/1, data_buffer1/3
  Delay76/1 -> Delay77/1, Inverter12/1, data_buffer2/3
  Delay77/1 -> Delay78/1, Inverter11/1, data_buffer3/3
  Delay78/1 -> Delay79/1, Inverter21/1, data_buffer4/3
  Delay79/1 -> Delay80/1, Inverter15/1, data_buffer5/3
  Delay80/1 -> Delay81/1, Inverter14/1, data_buffer6/3
  Delay81/1 -> Delay82/1, Inverter20/1, data_buffer7/3
  Delay82/1 -> Delay83/1, Inverter19/1, data_buffer8/3
  Delay83/1 -> Delay84/1, Inverter18/1, data_buffer9/3
  Delay85/1 -> Inverter22/1, data_buffer11/3
  Register13/1 -> [data1]
  Inverter16/1 -> Register13/2
  Register14/1 -> [data2]
  Inverter12/1 -> Register14/2
  Register15/1 -> [data3]
  Inverter11/1 -> Register15/2
  Register16/1 -> [data4]
  Inverter21/1 -> Register16/2
  Register17/1 -> [data5]
  Inverter15/1 -> Register17/2
  Register18/1 -> [data6]
  Inverter14/1 -> Register18/2
  Register19/1 -> [data7]
  Inverter20/1 -> Register19/2
  Register20/1 -> [data8]
  Inverter19/1 -> Register20/2
  Register21/1 -> [data9]
  Inverter18/1 -> Register21/2
  Register22/1 -> [data10]
  Inverter17/1 -> Register22/2
  Register23/1 -> [data11]
  Inverter22/1 -> Register23/2
  Delay43/1 -> pack_eof/1
  Delay48/1 -> Delay2/1
  Delay49/1 -> Delay48/1
  [eof] -> Delay49/1
  Delay53/1 -> [tx_header]
  data_buffer6/1 -> Register18/1
  Delay91/1 -> [header_end1]
  Delay92/1 -> [header_end2]
  Count_data7/1 -> Relational1/2
  [header_end1] -> Delay97/1, Register8/3, Register8/1, Count_data7/1
  Constant1/1 -> Relational1/1
  Relational1/1 -> Logical5/1
  Register8/1 -> Delay94/1
  Logical5/1 -> [start_read2], [start_read1]
  Delay94/1 -> Delay95/1, Logical5/2
  Delay95/1 -> Delay96/1
  Delay96/1 -> [read_en]
  Delay97/1 -> Delay98/1, Register8/2
  Delay98/1 -> Delay99/1
  Delay99/1 -> Delay100/1
  Delay100/1 -> Delay102/1
  Delay102/1 -> Delay103/1, Delay104/1, Delay105/1
  Delay103/1 -> [eof]
  Delay104/1 -> [eof_copy]
  Delay105/1 -> [eof_copy2]
  [header_end2] -> Register24/2
  data_buffer/1 -> Register12/1
  data_buffer1/1 -> Register13/1
  data_buffer2/1 -> Register14/1
  data_buffer3/1 -> Register15/1
  data_buffer4/1 -> Register16/1
  data_buffer5/1 -> Register17/1
  data_buffer11/1 -> Register23/1
  data_buffer7/1 -> Register19/1
  data_buffer8/1 -> Register20/1
  data_buffer9/1 -> Register21/1
  data_buffer10/1 -> Register22/1

== system eovsa_corr_300mhz/packetizer_x1 ==
  note: Use acc_num from P packetizer
  note: rst goes low
      | the clock after new_acc,
      | so any counters enabled
      | by new_acc
      | increment on the second pulse
  note: rst is high during first new_acc
  note: HACK!
  rst : Inport
  acc_data : Inport  Port=2
  acc_valid : Inport  Port=3
  acc_len : Inport  Port=4
  use_circular : Inport  Port=5
  x_eng_id : Inport  Port=6
  mcnt : Inport  Port=7
  new_acc : Inport  Port=8
  2x4byte_endian_flip : Subsystem
  Concat : xbsIndex_r4/Concat  num_inputs=3  dbl_ovrd=off  block_type=concat
  Convert3 : xbsIndex_r4/Convert  gui_display_data_type=Fixed-point  arith_type=Unsigned  n_bits=n_x  bin_pt=0  float_type=Single  exp_bits=8  fraction_bits=24  quantization=Truncate  overflow=Wrap  en=off  latency=0  dbl_ovrd=off  pipeline=off  block_type=convert
      settings: block_version=11.4
  Delay{1,7..8,11} (4 alike) : xbsIndex_r4/Delay  rst=off  infoeditControl=Selection of Reset will increase slice count due to use of real FFs and instead of SRLs  en=off  latency=1  dbl_ovrd=off  reg_retiming=off  block_type=delay
      settings: block_version=11.4
  Delay12 : xbsIndex_r4/Delay  rst=off  infoeditControl=Selection of Reset will increase slice count due to use of real FFs and instead of SRLs  en=off  latency=header_len / 8 + 1  dbl_ovrd=off  reg_retiming=on  block_type=delay
      settings: block_version=11.4
  Delay13 : xbsIndex_r4/Delay  rst=off  infoeditControl=Selection of Reset will increase slice count due to use of real FFs and instead of SRLs  en=off  latency=header_len / 8 + 1 - 1  dbl_ovrd=off  reg_retiming=on  block_type=delay
      settings: block_version=11.4
  Delay{4..6,14,20} (5 alike) : xbsIndex_r4/Delay  rst=off  infoeditControl=Selection of Reset will increase slice count due to use of real FFs and instead of SRLs  en=off  latency=1  dbl_ovrd=off  reg_retiming=on  block_type=delay
      settings: block_version=11.4
  Inverter : xbsIndex_r4/Inverter  en=off  latency=0  dbl_ovrd=off  block_type=inv
  Logical : xbsIndex_r4/Logical  logical_function=AND  inputs=2  en=off  latency=0  precision=Full  arith_type=Unsigned  n_bits=16  bin_pt=0  align_bp=on  dbl_ovrd=off  block_type=logical
  Mux3 : xbsIndex_r4/Mux  inputs=12  en=off  latency=1  precision=Full  arith_type=Unsigned  n_bits=16  bin_pt=14  quantization=Truncate  overflow=Wrap  dbl_ovrd=off  block_type=mux
      settings: block_version=11.4
  Register{,2..4} (4 alike) : xbsIndex_r4/Register  init=0  rst=on  en=on  dbl_ovrd=off  block_type=register
  Register1 : xbsIndex_r4/Register  init=0  rst=off  en=on  dbl_ovrd=off  block_type=register
  Register5 : xbsIndex_r4/Register  init=0  rst=off  en=on  dbl_ovrd=off  block_type=register
  Slice : xbsIndex_r4/Slice  nbits=2  boolean_output=off  mode=Lower Bit Location + Width  bit1=0  base1=MSB of Input  bit0=0  base0=LSB of Input  dbl_ovrd=off  block_type=slice
  Slice1 : xbsIndex_r4/Slice  nbits=log2(n_packets) - 2  boolean_output=off  mode=Lower Bit Location + Width  bit1=0  base1=MSB of Input  bit0=2  base0=LSB of Input  dbl_ovrd=off  block_type=slice
  count_accs : xbsIndex_r4/Counter  cnt_type=Free Running  cnt_to=50 - 1  operation=Up  start_count=0  cnt_by_val=1  arith_type=Unsigned  n_bits=32  bin_pt=0  load_pin=off  rst=on  en=on  explicit_period=on  period=1  dbl_ovrd=off  use_behavioral_HDL=off  implementation=DSP48  use_rpm=off  block_type=counter
  count_header : xbsIndex_r4/Counter  cnt_type=Count Limited  cnt_to=header_len / 8 - 1 + 1  operation=Up  start_count=0  cnt_by_val=1  arith_type=Unsigned  n_bits=ceil( log2( header_len / 8 - 1 + 1) )  bin_pt=0  load_pin=off  rst=on  en=on  explicit_period=on  period=1  dbl_ovrd=off  use_behavioral_HDL=on  implementation=Fabric  use_rpm=off  block_type=counter
  count_packets : xbsIndex_r4/Counter  cnt_type=Count Limited  cnt_to=n_packets - 1  operation=Up  start_count=0  cnt_by_val=1  arith_type=Unsigned  n_bits=ceil( log2( n_packets ) )  bin_pt=0  load_pin=off  rst=on  en=on  explicit_period=off  period=1  dbl_ovrd=off  use_behavioral_HDL=on  implementation=Fabric  use_rpm=off  block_type=counter
  count_seconds : xbsIndex_r4/Counter  cnt_type=Count Limited  cnt_to=50 - 1  operation=Up  start_count=0  cnt_by_val=1  arith_type=Unsigned  n_bits=ceil(log2(50))  bin_pt=0  load_pin=off  rst=on  en=on  explicit_period=on  period=1  dbl_ovrd=off  use_behavioral_HDL=on  implementation=Fabric  use_rpm=off  block_type=counter
  edge_detect : Subsystem  AncestorBlock=casper_library_misc/edge_detect  mask(edge_detect){edge=Falling, polarity=Active High, x_in=[0 0.08 0.08 0.16 0.16 0.24 0.24 0.32 0.32 0.4], y_in=[-1 -1  1  1  1  1  1  1  1  1], x_out=[0.6 0.68 0.68 0.76 0.76 0.84 0.84 0.92 0.92 1], y_out=[-1 -1  1  1 -1 -1 -1 -1 -1 -1]}
      mask prompts: edge "Edge Type"; polarity "Output Polarity"; x_in "Input X Positions"; y_in "Input Y Positions"; x_out "Output X Positions"; y_out "Output Y Positions"
      mask help: Output is active for one-cycle after each edge of the specified type (i.e. rising, falling or both).
      mask init: same as eovsa_corr_300mhz/edge_detect1
      settings: AttributesFormatString=|
      | falling edges
      | active high
      mask Help: Output is active for one-cycle after each edge of the specified type (i.e. rising, falling, or both).  Latency is zero.
      mask TypeOptions edge: Rising | Falling | Both
      mask TypeOptions polarity: Active High | Active Low
      mask Display:
      | plot(x_in_num,0.5+y_in_num*0.2);
      | plot(x_out_num,0.5+y_out_num*0.2);
  edge_detect2 : Subsystem  AncestorBlock=casper_library_misc/edge_detect  mask(edge_detect){edge=Rising, polarity=Active High, x_in=[0 0.08 0.08 0.16 0.16 0.24 0.24 0.32 0.32 0.4], y_in=[-1 -1  1  1  1  1  1  1  1  1], x_out=[0.6 0.68 0.68 0.76 0.76 0.84 0.84 0.92 0.92 1], y_out=[-1 -1  1  1 -1 -1 -1 -1 -1 -1]}
      mask prompts: edge "Edge Type"; polarity "Output Polarity"; x_in "Input X Positions"; y_in "Input Y Positions"; x_out "Output X Positions"; y_out "Output Y Positions"
      mask help: Output is active for one-cycle after each edge of the specified type (i.e. rising, falling or both).
      mask init: same as eovsa_corr_300mhz/edge_detect1
      settings: AttributesFormatString=|
      | rising edges
      | active high
      mask Help: Output is active for one-cycle after each edge of the specified type (i.e. rising, falling, or both).  Latency is zero.
      mask TypeOptions edge: Rising | Falling | Both
      mask TypeOptions polarity: Active High | Active Low
      mask Display:
      | plot(x_in_num,0.5+y_in_num*0.2);
      | plot(x_out_num,0.5+y_out_num*0.2);
  header_x : Subsystem
  massage : Subsystem
  pulse_ext : casper_library_misc/pulse_ext  pulse_len=header_len / 8
      link override Constant5: const=pulse_len  gui_display_data_type=Fixed-point  arith_type=Unsigned  n_bits=bits  bin_pt=0  preci_type=Single  exp_width=8  frac_width=24  explicit_period=off  period=1  equ=P=C  opselect=C  inp2=PCIN>>17  opr=+  inp1=P  carry=CIN  dbl_ovrd=off
  pulse_ext1 : casper_library_misc/pulse_ext  pulse_len=(header_len +payload_bytes) / 8
  pack_data : Outport
  data_valid : Outport  Port=2
  pack_eof : Outport  Port=3
  wires:
  2x4byte_endian_flip/1(Out1) -> Delay12/1
  Register5/1 -> header_x/5(acc_num_pps)
  count_seconds/1 -> Register5/1
  Delay8/1 -> Register3/2
  Delay7/1 -> Register/2, Delay8/1
  [new_acc] -> count_seconds/2, Register5/2
  [new_acc] -> count_accs/2
  Register3/1 -> [acc_num]
  acc_data/1 -> 2x4byte_endian_flip/1(In1)
  Inverter/1 -> [rst]
  Delay1/1 -> Register/3, Register3/3
  [acc_num] -> header_x/3(acc_num)
  [new_acc] -> Delay1/1
  [acc_num_P] -> Register/1
  [rst] -> Delay7/1
  Register/1 -> Register3/1
  Register4/1 -> Inverter/1
  [new_acc] -> Register4/1, Register4/3
  [rst] -> count_accs/1
  [rst] -> count_seconds/1
  Slice1/1 -> Concat/3
  Slice/1 -> Concat/2
  [mcnt_this_packet] -> header_x/8(mcnt)
  massage/1(Out1) -> header_x/2(acc_len)
  acc_len/1 -> massage/1(In1)
  [eof] -> Delay13/1
  count_header/1 -> Mux3/1
  Logical/1 -> data_valid/1
  Delay6/1 -> Logical/1
  Register2/1 -> Logical/2
  rst/1 -> Register2/2, Register4/2
  Delay4/1 -> pack_eof/1
  Delay20/1 -> Delay6/1, Register2/1, Register2/3
  pulse_ext1/1 -> Delay20/1
  [new_packet] -> pulse_ext1/1
  Delay14/1 -> Delay4/1
  Delay13/1 -> Delay14/1
  Delay12/1 -> Mux3/13
  pulse_ext/1 -> count_header/2
  [new_packet] -> count_header/1, pulse_ext/1
  Delay11/1 -> Register1/2
  Register1/1 -> [mcnt_this_packet]
  [new_acc] -> Delay11/1
  mcnt/1 -> Register1/1
  edge_detect2/1(out) -> [new_packet]
  [eof] -> count_packets/2
  [new_acc] -> count_packets/1
  new_acc/1 -> [new_acc]
  edge_detect/1(out) -> [eof]
  acc_valid/1 -> edge_detect/1(in), edge_detect2/1(in)
  Mux3/1 -> Delay5/1
  count_packets/1 -> header_x/1(packet_num), Slice1/1, Slice/1
  use_circular/1 -> header_x/6(circular)
  header_x/1(header0) -> Mux3/2
  header_x/2(header1) -> Mux3/3
  header_x/3(header2) -> Mux3/4
  header_x/4(header3) -> Mux3/5
  header_x/5(header4) -> Mux3/6
  header_x/6(header5) -> Mux3/7
  header_x/7(header6) -> Mux3/8
  header_x/8(header7) -> Mux3/9
  header_x/9(header8) -> Mux3/10
  header_x/10(header9) -> Mux3/11
  header_x/11(header10) -> Mux3/12
  x_eng_id/1 -> Convert3/1, header_x/4(xeng_id)
  Concat/1 -> header_x/7(subband_index)
  Delay5/1 -> pack_data/1
  Convert3/1 -> Concat/1
